simulink model "LQR"  (R2016a)
settings: Solver=VariableStepAuto  StartTime=0.0  StopTime=5  RelTol=1e-3
values from neighbouring files (symbols this model uses):
  A = [0.8978 1.6108 0 0; 0 0 0.2237 -17.695; 0 0 -2.2649 1231.1; 0 0 -0.0063 0]    [LQR1.m]    (also in LQR2.m = [0.8978-0.3416 1.6108-0.4431 0 0  ;0 0 0.2237-0.0318 -17.695; controlability_check.m)
  B = [ 114.35; 38.942; 0; -2.3455]    [LQR1.m]    (also in LQR2.m = [114.35 ;38.942;0;-2.3455 ]; controlability_check.m)
  k1 = K(1)    [LQR2.m]
  k2 = K(2)    [LQR2.m]
  k3 = K(3)    [LQR2.m]
  k4 = K(4)    [LQR2.m]
settings Model: Creator=Shrouk  LastModifiedBy=Shrouk

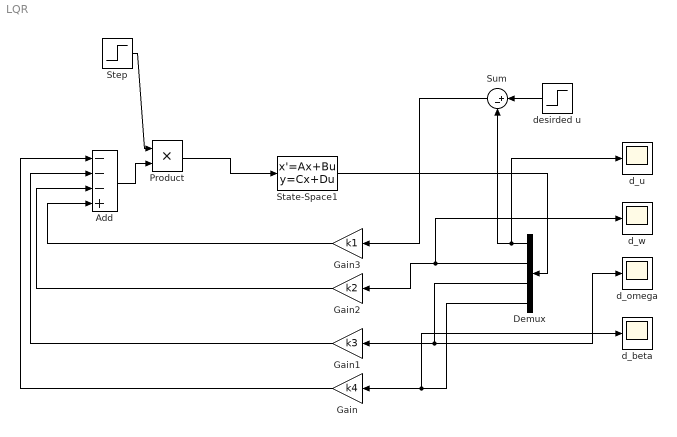
== system LQR ==
  " d_u " : Scope
  Add : Sum  Inputs=---+
  Demux : Demux
  Gain : Gain  Gain=k4
  Gain1 : Gain  Gain=k3
  Gain2 : Gain  Gain=k2
  Gain3 : Gain  Gain=k1
  Product : Product
  State-Space1 : StateSpace  A=A  B=B  C=eye(4)  D=[0;0;0;0]  X0=0
  Step : Step  SampleTime=0
  Sum : Sum  Inputs=|+-
  d_beta : Scope
  d_omega : Scope
  d_w : Scope
  desirded u : Step  After=4  SampleTime=0
  wires:
  State-Space1/1 -> Demux/1
  Gain2/1 -> Add/3
  Gain1/1 -> Add/2
  Gain/1 -> Add/1
  Demux/1 -> " d_u "/1, Sum/2
  Demux/2 -> d_w/1, Gain2/1
  Demux/3 -> Gain1/1, d_omega/1
  Demux/4 -> d_beta/1, Gain/1
  desirded u/1 -> Sum/1
  Sum/1 -> Gain3/1
  Step/1 -> Product/1
  Add/1 -> Product/2
  Product/1 -> State-Space1/1
  Gain3/1 -> Add/4
